simulink model "controller"  (R2020a)
settings: Solver=FixedStepDiscrete  StartTime=0.0  StopTime=10.0  FixedStep=0.01  MaxStep=0.01  RelTol=1e-3
undefined symbols (not defined in the file): DiscIntNeverNeededParam
libraries: dspfdesign x2, powerlib_meascontrol x2, simulink x2, dspswit3 x1, dspsigattribs x1
Description:
  | Ventilator Controller
settings Model: Creator=upattacini  LastModifiedBy=upattacini
settings SolverCC: MaxConsecutiveMinStep=10
settings DataIOCC: SaveOutput=off  SignalLogging=off  DSMLogging=off  SaveTime=off  ReturnWorkspaceOutputs=off
settings OptimizationCC: DefaultUnderspecifiedDataType=single  StrengthReduction=on  ZeroExternalMemoryAtStartup=off  ZeroInternalMemoryAtStartup=off  OptimizeBlockOrder=speed  OptimizationPriority=Speed  OptimizationCustomize=off  MultiThreadedLoops=on  EfficientTunableParamExpr=on
settings DebuggingCC: ParameterTunabilityLossMsg=error
settings SFSimCC: MATLABDynamicMemAlloc=off
settings RTWCC: SystemTargetFile=ert.tlc  GenCodeOnly=on  PackageGeneratedCodeAndArtifacts=on  PackageName=controller  TemplateMakefile=ert_default_tmf  TargetLang=C++
settings CodeAppCC: ForceParamTrailComments=on  IgnoreCustomStorageClasses=off  OperatorAnnotations=on  SimulinkDataObjDesc=on  SFDataObjDesc=on  InsertBlockDesc=on
settings ERTTargetCC: TargetLangStandard=C++03 (ISO)  GenerateSampleERTMain=on  MultiInstanceERTCode=on  CodeInterfacePackaging=C++ class  RootIOFormat=Structure reference  ERTCustomFileTemplate=example_file_process.tlc

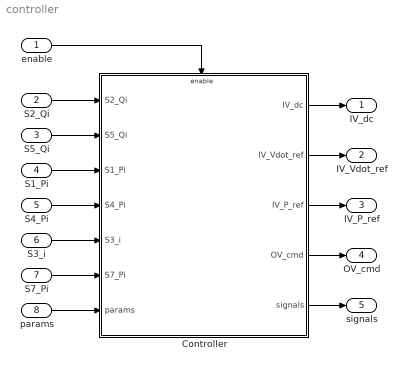
== system controller ==
  enable : Inport  OutDataTypeStr=boolean
  S2_Qi : Inport  Port=2  OutDataTypeStr=single
  S5_Qi : Inport  Port=3  OutDataTypeStr=single
  S1_Pi : Inport  Port=4  OutDataTypeStr=single
  S4_Pi : Inport  Port=5  OutDataTypeStr=single
  S3_i : Inport  Port=6  OutDataTypeStr=single  PortDimensions=2
  S7_Pi : Inport  Port=7  OutDataTypeStr=single
  params : Inport  Port=8  OutDataTypeStr=single  PortDimensions=3
  Controller : Subsystem  Tag=PublishSubsystem  mask(Controller){control_mode=PRESSURE, tidal_volume=0.65, PIP=35, PIP_step_perc=75, PIP_rise_perc=70, PEEP=5, respiratory_rate=10, IE_ratio=1/2, VC_P=0.2, VC_I=10, PC_FFW=30, PC_P=1, PC_I=40, HSC_cutoff=25, enable_trigger=off, trigger_inhibition_time=0.5, trigger_cutoff=2.5, trigger_filtder_tau=0.1, trigger_hyst_up=-5, trigger_hyst_down=-10}
      mask prompts: control_mode "Control Mode"; tidal_volume "Tidal Volume (L)"; PIP "PIP (cmH2O)"; PIP_step_perc "PIP Step Percentage (%)"; PIP_rise_perc "PIP Rising Percentage (%)"; PEEP "PEEP (cmH2O)"; respiratory_rate "Respiratory Rate (breaths/min)"; IE_ratio "Inspiration to Expiration Ratio"; VC_P "Proportional (%FS/SLPM)"; VC_I "Integral (%FS/(SLPM*s))"; PC_FFW "Feed-Forward (%FS)"; PC_P "Proportional (%FS/cmH2O)"; PC_I "Integral (%FS/(cmH2O*s))"; HSC_cutoff "HSC Cutoff Frequency (Hz)"; enable_trigger "Enable Triggering"; trigger_inhibition_time "Inhibition Time (s)"; trigger_cutoff "S3 Cutoff Frequency (Hz)"; trigger_filtder_tau "Derivative Filter Time Constant (s)"; trigger_hyst_up "Hysteresis Threshold Up (cmH2O/s)"; trigger_hyst_down "Hysteresis Threshold Down (cmH2O/s)"
      mask help: The controller generates the input signals that controls the inspiratory flow and expiratory valve.
      mask init:
      | Ts = eval(get_param(gcs, 'FixedStep'));
      | 
      | VC_mode = control_mode == 2;
      | PC_mode = control_mode == 3;
      | 
      | PC_IST = (IE_ratio/(IE_ratio+1) * (60 / respiratory_rate)) * (PIP_rise_perc/100) / 1.5;
      | a = -150.7658/(PC_IST*PC_IST*PC_IST);
      | b = -84.98128/(PC_IST*PC_IST);
      | c = -15.96696/PC_IST;
      | 
      | m = 4.0*c*Ts;
      | n = 2.0*b*Ts*Ts;
      | p = a*Ts*Ts*Ts;
      | 
      | PC_IST_num = [p, 3*p, 3*p, p];
      | PC_IST_den = [m+n+p-8, -m+n+3*p+24, -m-n+3*p-24, m-n+p+8];
      | PC_IST_x0_Gain = (PC_IST_den(2) - PC_IST_num(1)) / ...
      |                  ( PC_IST_num(2)*sum(PC_IST_den(2:end)) + ...
      |                  PC_IST_den(2)*sum(PC_IST_num(2:end)) );
      mask TypeOptions control_mode: OFF | VOLUME | PRESSURE
      mask Callback control_mode:
      | numparams = Simulink.Mask.get(gcb).numParameters;
      | enable = cell(1, numparams);
      | enable(:) = {'on'};
      | 
      | control_mode = get_param(gcb, 'control_mode');
      | if strcmpi(control_mode, 'VOLUME')
      |     enable(3:5) = {'off'};
      |     enable(11:13) = {'off'};
      | elseif strcmpi(control_mode, 'PRESSURE')
      |     enable{2} = 'off';
      |     enable(9:10) = {'off'};
      | else
      |     enable(2:end-6) = {'off'};
      |     enable(end-4:end) = {'off'};
      | end
      | set_param(gcb, 'MaskEnables', enable);
      mask DialogControl Container2 Prompt: Medical Parameters
      mask DialogControl Container3 Prompt: Controller Parameters
      mask DialogControl Container4 Prompt: Volume Control
      mask DialogControl Container5 Prompt: Pressure Control
      mask DialogControl Container6 Prompt: Filtering
      mask DialogControl Container7 Prompt: Assisted Ventilation
  IV_dc : Outport
  IV_Vdot_ref : Outport  Port=2
  IV_P_ref : Outport  Port=3
  OV_cmd : Outport  Port=4
  signals : Outport  Port=5
  wires:
  S2_Qi/1 -> Controller/1(S2_Qi)
  Controller/1(IV_dc) -> IV_dc/1
  Controller/2(IV_Vdot_ref) -> IV_Vdot_ref/1
  Controller/4(OV_cmd) -> OV_cmd/1
  S1_Pi/1 -> Controller/3(S1_Pi)
  Controller/3(IV_P_ref) -> IV_P_ref/1
  Controller/5(signals) -> signals/1
  enable/1 -> Controller/Enable
  S5_Qi/1 -> Controller/2(S5_Qi)
  S4_Pi/1 -> Controller/4(S4_Pi)
  params/1 -> Controller/7(params)
  S3_i/1 -> Controller/5(S3_i)
  S7_Pi/1 -> Controller/6(S7_Pi)

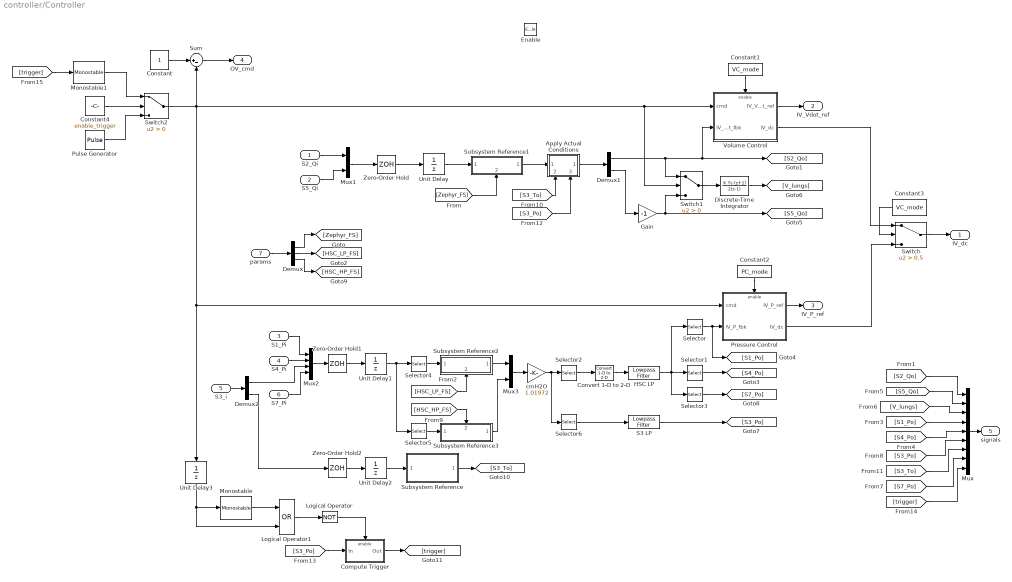
== system controller/Controller ==
  S2_Qi : Inport
  S5_Qi : Inport  Port=2
  S1_Pi : Inport  Port=3
  S4_Pi : Inport  Port=4
  S3_i : Inport  Port=5
  S7_Pi : Inport  Port=6
  params : Inport  Port=7
  Enable : EnablePort  StatesWhenEnabling=reset
  Apply Actual Conditions : Subsystem  ReferencedSubsystem=apply_actual_conditions
      settings: PortSchema="{\"entries\":[{\"content\":{\"sides\":[{\"content\":{\"connectorIds\":[\"In1\"]},\"type\":\"ConnectorPlacement.EquallySpacedRectSide\",\"uuid\":\"3b4e15f5-ec7a-455d-a112-e063b421ee9f\"},{\"content\":{\"connectorIds\":[\"Out1\"],\"side\":\"RIGHT\"},\"type\":\"ConnectorPlacement.EquallySpacedRectSide\",\"uuid\":\"595b3fd5-6603-4191-b183-4edf5336d9a2\"},{\"content\":{\"connectorIds\":[],\"side\":\"TOP\"},\"type\":\"ConnectorPlacement.EquallySpacedRectSide\",\"uuid\":\"7211f4ea-7225-4536-b1e6-5aea95971c19\"},{\"content\":{\"connectorIds\":[\"In2\",\"In3\"],\"side\":\"BOTTOM\"},\"type\":\"ConnectorPlacement.EquallySpacedRectSide\",\"uuid\":\"c060314b-2654-4a54-a68c-60767f6efbb5\"}]},\"type\":\"ConnectorPlacement.EquallySpacedConnector\",\"uuid\":\"0e2934c3-16fd-4aed-85e0-c12757e58969\"}],\"packageUris\":[\"http://schema.mathworks.com/mf0/Connector/19700101\"],\"version\":\"1.0\"}"
  Compute Trigger : Subsystem
  Constant : Constant  OutDataTypeStr=single
  Constant1 : Constant  Value=VC_mode
  Constant2 : Constant  Value=PC_mode
  Constant3 : Constant  Value=VC_mode
  Constant4 : Constant  Value=enable_trigger  OutDataTypeStr=boolean
  Convert 1-D to 2-D : dspsigattribs/Convert 1-D to 2-D  M=1  N=3  frameBasedOut=off
      settings: SourceProductBaseCode=DS
  Demux : Demux  Outputs=3
  Demux1 : Demux  Outputs=2
  Demux2 : Demux  Outputs=2
  Discrete-Time Integrator : DiscreteIntegrator  IntegratorMethod=Integration: Trapezoidal  gainval=1/60  SampleTime=-1  ICPrevOutput=DiscIntNeverNeededParam  ICPrevScaledInput=DiscIntNeverNeededParam
  Gain : Gain  Gain=-1
  HSC LP : dspfdesign/Lowpass Filter  FilterType=IIR  DesignForMinimumOrder=off  FilterOrder=3  PassbandFrequency=HSC_cutoff  StopbandFrequency=12e3  PassbandRipple=0.5  StopbandAttenuation=30  InheritSampleRate=on  SampleRate=44100  SimulateUsing=Code generation  roundingMode=Floor  coeffsDataTypeStr=fixdt(1,16)
  Logical Operator : Logic  Operator=NOT  AllPortsSameDT=off  OutDataTypeStr=boolean
  Logical Operator1 : Logic  Operator=OR  AllPortsSameDT=off  OutDataTypeStr=boolean
  Monostable : powerlib_meascontrol/Logic/Monostable  EdgeDetect=Falling  PulseDuration=trigger_inhibition_time  ic=0  Ts=Ts
      settings: SourceProductBaseCode=PS
  Monostable1 : powerlib_meascontrol/Logic/Monostable  EdgeDetect=Rising  PulseDuration=IE_ratio/(IE_ratio+1) * (60 / respiratory_rate)  ic=0  Ts=Ts
      settings: SourceProductBaseCode=PS
  Mux : Mux  Inputs=9
  Mux1 : Mux  Inputs=2
  Mux2 : Mux
  Mux3 : Mux  Inputs=2
  Pressure Control : Subsystem
  Pulse Generator : DiscretePulseGenerator  Period=floor((60 / respiratory_rate) / Ts)  PulseWidth=floor((IE_ratio/(IE_ratio+1) * (60 / respiratory_rate)) / Ts)  SampleTime=Ts
  S3 LP : dspfdesign/Lowpass Filter  FilterType=IIR  DesignForMinimumOrder=off  FilterOrder=3  PassbandFrequency=trigger_cutoff  StopbandFrequency=12e3  PassbandRipple=0.5  StopbandAttenuation=30  InheritSampleRate=on  SampleRate=44100  SimulateUsing=Code generation  roundingMode=Floor  coeffsDataTypeStr=fixdt(1,16)
  Selector : Selector  InputPortWidth=3  IndexOptions=Index vector (dialog)  Indices=1  OutputSizes=1
  Selector1 : Selector  InputPortWidth=3  IndexOptions=Index vector (dialog)  Indices=2  OutputSizes=1
  Selector2 : Selector  InputPortWidth=4  IndexOptions=Index vector (dialog)  Indices=[1 2 4]  OutputSizes=1
  Selector3 : Selector  InputPortWidth=3  IndexOptions=Index vector (dialog)  Indices=3  OutputSizes=1
  Selector4 : Selector  InputPortWidth=4  IndexOptions=Index vector (dialog)  Indices=[1 2 3]  OutputSizes=1
  Selector5 : Selector  InputPortWidth=4  IndexOptions=Index vector (dialog)  Indices=4  OutputSizes=1
  Selector6 : Selector  InputPortWidth=4  IndexOptions=Index vector (dialog)  Indices=3  OutputSizes=1
  Subsystem Reference : Subsystem  ReferencedSubsystem=T_decoder
  Subsystem Reference1 : Subsystem  ReferencedSubsystem=HSC_decoder
      settings: PortSchema="{\"entries\":[{\"content\":{\"sides\":[{\"content\":{\"connectorIds\":[\"In1\"]},\"type\":\"ConnectorPlacement.EquallySpacedRectSide\",\"uuid\":\"71a4e4f9-9ef6-4add-947e-0b57a706a0fc\"},{\"content\":{\"connectorIds\":[\"Out1\"],\"side\":\"RIGHT\"},\"type\":\"ConnectorPlacement.EquallySpacedRectSide\",\"uuid\":\"d997839f-7697-403c-ab31-97bb95e5d26f\"},{\"content\":{\"connectorIds\":[],\"side\":\"TOP\"},\"type\":\"ConnectorPlacement.EquallySpacedRectSide\",\"uuid\":\"6a2eaf4c-1277-4d90-b513-5efc8abce9b0\"},{\"content\":{\"connectorIds\":[\"In2\"],\"side\":\"BOTTOM\"},\"type\":\"ConnectorPlacement.EquallySpacedRectSide\",\"uuid\":\"a341bd79-bd1c-4a8b-9abf-5623b4073918\"}]},\"type\":\"ConnectorPlacement.EquallySpacedConnector\",\"uuid\":\"c1361fad-ebea-4dab-bf9b-dc7c859591e9\"}],\"packageUris\":[\"http://schema.mathworks.com/mf0/Connector/19700101\"],\"version\":\"1.0\"}"
  Subsystem Reference2 : Subsystem  ReferencedSubsystem=HSC_decoder
      settings: PortSchema="{\"entries\":[{\"content\":{\"sides\":[{\"content\":{\"connectorIds\":[\"In1\"]},\"type\":\"ConnectorPlacement.EquallySpacedRectSide\",\"uuid\":\"71a4e4f9-9ef6-4add-947e-0b57a706a0fc\"},{\"content\":{\"connectorIds\":[\"Out1\"],\"side\":\"RIGHT\"},\"type\":\"ConnectorPlacement.EquallySpacedRectSide\",\"uuid\":\"d997839f-7697-403c-ab31-97bb95e5d26f\"},{\"content\":{\"connectorIds\":[],\"side\":\"TOP\"},\"type\":\"ConnectorPlacement.EquallySpacedRectSide\",\"uuid\":\"6a2eaf4c-1277-4d90-b513-5efc8abce9b0\"},{\"content\":{\"connectorIds\":[\"In2\"],\"side\":\"BOTTOM\"},\"type\":\"ConnectorPlacement.EquallySpacedRectSide\",\"uuid\":\"a341bd79-bd1c-4a8b-9abf-5623b4073918\"}]},\"type\":\"ConnectorPlacement.EquallySpacedConnector\",\"uuid\":\"c1361fad-ebea-4dab-bf9b-dc7c859591e9\"}],\"packageUris\":[\"http://schema.mathworks.com/mf0/Connector/19700101\"],\"version\":\"1.0\"}"
  Subsystem Reference3 : Subsystem  ReferencedSubsystem=HSC_decoder
      settings: PortSchema="{\"entries\":[{\"content\":{\"sides\":[{\"content\":{\"connectorIds\":[\"In1\"]},\"type\":\"ConnectorPlacement.EquallySpacedRectSide\",\"uuid\":\"71a4e4f9-9ef6-4add-947e-0b57a706a0fc\"},{\"content\":{\"connectorIds\":[\"Out1\"],\"side\":\"RIGHT\"},\"type\":\"ConnectorPlacement.EquallySpacedRectSide\",\"uuid\":\"d997839f-7697-403c-ab31-97bb95e5d26f\"},{\"content\":{\"connectorIds\":[\"In2\"],\"side\":\"TOP\"},\"type\":\"ConnectorPlacement.EquallySpacedRectSide\",\"uuid\":\"6a2eaf4c-1277-4d90-b513-5efc8abce9b0\"},{\"content\":{\"connectorIds\":[],\"side\":\"BOTTOM\"},\"type\":\"ConnectorPlacement.EquallySpacedRectSide\",\"uuid\":\"a341bd79-bd1c-4a8b-9abf-5623b4073918\"}]},\"type\":\"ConnectorPlacement.EquallySpacedConnector\",\"uuid\":\"c1361fad-ebea-4dab-bf9b-dc7c859591e9\"}],\"packageUris\":[\"http://schema.mathworks.com/mf0/Connector/19700101\"],\"version\":\"1.0\"}"
  Sum : Sum  Inputs=|+-
  Switch : Switch  Criteria=u2 > Threshold  Threshold=0.5
  Switch1 : Switch  Criteria=u2 > Threshold
  Switch2 : Switch  Criteria=u2 > Threshold  OutDataTypeStr=single
  Unit Delay : UnitDelay  SampleTime=-1  HasFrameUpgradeWarning=on
  Unit Delay1 : UnitDelay  InitialCondition=0.1 * 16384  SampleTime=-1  HasFrameUpgradeWarning=on
  Unit Delay2 : UnitDelay  SampleTime=-1  HasFrameUpgradeWarning=on
  Unit Delay3 : UnitDelay  SampleTime=-1  HasFrameUpgradeWarning=on
  Volume Control : Subsystem
  Zero-Order Hold : ZeroOrderHold  SampleTime=Ts
  Zero-Order Hold1 : ZeroOrderHold  SampleTime=Ts
  Zero-Order Hold2 : ZeroOrderHold  SampleTime=Ts
  cmH2O : Gain  Gain=1.01972
  IV_dc : Outport  OutputWhenDisabled=reset  InitialOutput=0
  IV_Vdot_ref : Outport  Port=2  OutputWhenDisabled=reset  InitialOutput=0
  IV_P_ref : Outport  Port=3  OutputWhenDisabled=reset  InitialOutput=0
  OV_cmd : Outport  Port=4  OutputWhenDisabled=reset  InitialOutput=0
  signals : Outport  Port=5  OutputWhenDisabled=reset  InitialOutput=0
  wires:
  Constant/1 -> Sum/1
  Sum/1 -> OV_cmd/1
  Volume Control/1(IV_Vdot_ref) -> IV_Vdot_ref/1
  Constant1/1 -> Volume Control/Enable
  Constant2/1 -> Pressure Control/Enable
  Switch/1 -> IV_dc/1
  Volume Control/2(IV_dc) -> Switch/1
  Pressure Control/2(IV_dc) -> Switch/3
  Constant3/1 -> Switch/2
  Pressure Control/1(IV_P_ref) -> IV_P_ref/1
  params/1 -> Demux/1
  Demux/1 -> [Zephyr_FS]
  [Zephyr_FS] -> Subsystem Reference1/2
  [S2_Qo] -> Mux/1
  Mux/1 -> signals/1
  Zero-Order Hold/1 -> Unit Delay/1
  Zero-Order Hold1/1 -> Unit Delay1/1
  Unit Delay1/1 -> Selector5/1, Selector4/1
  Demux/2 -> [HSC_LP_FS]
  [HSC_LP_FS] -> Subsystem Reference2/2
  [S5_Qo] -> Mux/2
  Gain/1 -> Switch1/3, [S5_Qo]
  [S1_Po] -> Mux/4
  [S4_Po] -> Mux/5
  Discrete-Time Integrator/1 -> [V_lungs]
  [V_lungs] -> Mux/3
  [S3_Po] -> Mux/6
  S2_Qi/1 -> Mux1/1
  S5_Qi/1 -> Mux1/2
  Mux1/1 -> Zero-Order Hold/1
  S4_Pi/1 -> Mux2/2
  Mux2/1 -> Zero-Order Hold1/1
  Convert 1-D to 2-D/1 -> HSC LP/1
  Selector/1 -> [S1_Po], Pressure Control/2(IV_P_fbk)
  HSC LP/1 -> Selector3/1, Selector1/1, Selector/1
  Selector1/1 -> [S4_Po]
  S7_Pi/1 -> Mux2/4
  Selector3/1 -> [S7_Po]
  Demux/3 -> [HSC_HP_FS]
  Selector4/1 -> Subsystem Reference2/1
  Selector5/1 -> Subsystem Reference3/1
  [HSC_HP_FS] -> Subsystem Reference3/2
  Subsystem Reference2/1 -> Mux3/1
  Subsystem Reference3/1 -> Mux3/2
  Mux3/1 -> cmH2O/1
  S1_Pi/1 -> Mux2/1
  Demux2/1 -> Mux2/3
  [S7_Po] -> Mux/8
  Demux2/2 -> Zero-Order Hold2/1
  S3_i/1 -> Demux2/1
  Demux1/1 -> Switch1/1, Volume Control/2(IV_Vdot_fbk), [S2_Qo]
  Demux1/2 -> Gain/1
  Unit Delay2/1 -> Subsystem Reference/1
  [S3_To] -> Mux/7
  Zero-Order Hold2/1 -> Unit Delay2/1
  Subsystem Reference/1 -> [S3_To]
  [S3_To] -> Apply Actual Conditions/2
  Unit Delay/1 -> Subsystem Reference1/1
  Subsystem Reference1/1 -> Apply Actual Conditions/1
  Apply Actual Conditions/1 -> Demux1/1
  Switch1/1 -> Discrete-Time Integrator/1
  [trigger] -> Mux/9
  Compute Trigger/1(Out) -> [trigger]
  Monostable/1 -> Logical Operator1/1
  Logical Operator1/1 -> Logical Operator/1
  Constant4/1 -> Switch2/2
  Pulse Generator/1 -> Switch2/3
  Logical Operator/1 -> Compute Trigger/Enable
  Unit Delay3/1 -> Logical Operator1/2, Monostable/1
  Monostable1/1 -> Switch2/1
  Switch2/1 -> Switch1/2, Volume Control/1(cmd), Pressure Control/1(cmd), Unit Delay3/1, Sum/2
  [trigger] -> Monostable1/1
  cmH2O/1 -> Selector6/1, Selector2/1
  [S3_Po] -> Apply Actual Conditions/3
  [S3_Po] -> Compute Trigger/1(In)
  Selector2/1 -> Convert 1-D to 2-D/1
  Selector6/1 -> S3 LP/1
  S3 LP/1 -> [S3_Po]

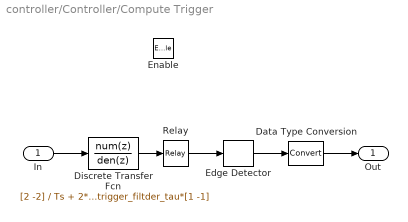
== system controller/Controller/Compute Trigger ==
  In : Inport
  Enable : EnablePort  StatesWhenEnabling=reset
  Data Type Conversion : DataTypeConversion
  Discrete Transfer Fcn : DiscreteTransferFcn  Numerator=[2 -2]  Denominator=Ts + 2*trigger_filtder_tau*[1 -1]
  Edge Detector : dspswit3/Edge Detector  InputProcessing=Columns as channels (frame based)
      settings: SourceProductBaseCode=DS
  Relay : Relay  OnSwitchValue=trigger_hyst_up  OffSwitchValue=trigger_hyst_down  OnOutputValue=0  OffOutputValue=1  OutDataTypeStr=Inherit: Inherit via back propagation
  Out : Outport  OutputWhenDisabled=reset  InitialOutput=0
  wires:
  Relay/1 -> Edge Detector/1
  Edge Detector/1 -> Data Type Conversion/1
  Data Type Conversion/1 -> Out/1
  Discrete Transfer Fcn/1 -> Relay/1
  In/1 -> Discrete Transfer Fcn/1

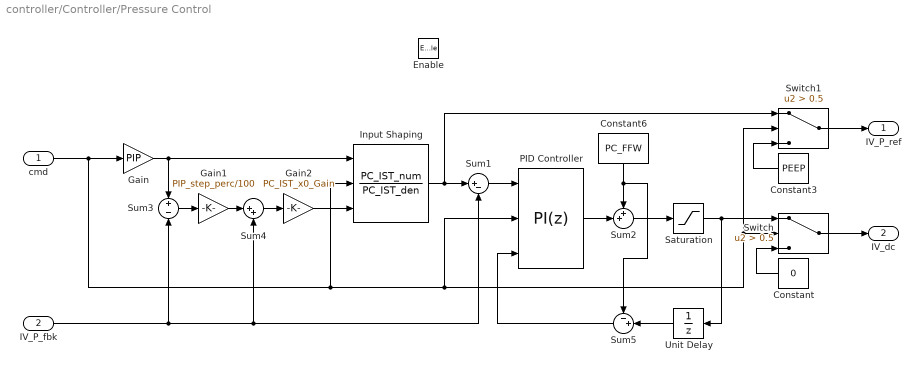
== system controller/Controller/Pressure Control ==
  cmd : Inport
  IV_P_fbk : Inport  Port=2
  Enable : EnablePort  StatesWhenEnabling=reset
  Constant : Constant  Value=0  OutDataTypeStr=single
  Constant3 : Constant  Value=PEEP  OutDataTypeStr=single
  Constant6 : Constant  Value=PC_FFW  OutDataTypeStr=single
  Gain : Gain  Gain=PIP
  Gain1 : Gain  Gain=PIP_step_perc/100
  Gain2 : Gain  Gain=PC_IST_x0_Gain
  Input Shaping : DiscreteFilter  Numerator=PC_IST_num  Denominator=PC_IST_den  InitialStatesSource=Input port  ExternalReset=Rising
      settings: InputPortMap=u0,r7,p5
  PID Controller : simulink/Continuous/PID Controller  Controller=PI  Form=Parallel  TimeDomain=Discrete-time  UseExternalTs=off  SampleTime=-1  IntegratorMethod=Trapezoidal  FilterMethod=Trapezoidal  ControllerParametersSource=internal  P=PC_P  I=PC_I  D=1  UseFilter=on  N=100  TunerSelectOption=Transfer Function Based (PID Tuner App)  InitialConditionSource=internal  InitialConditionForIntegrator=0  InitialConditionForFilter=0  DifferentiatorICPrevScaledInput=0  ExternalReset=rising  TrackingMode=on  Kt=1  LimitOutput=off  UpperSaturationLimit=100  LowerSaturationLimit=0  LinearizeAsGain=on  AntiWindupMode=clamping  Kb=1  POutMin=[]  POutMax=[]  IOutMin=[]  IOutMax=[]  DOutMin=[]  DOutMax=[]  NOutMin=[]  NOutMax=[]  SumOutMin=[]  SumOutMax=[]  SaturationOutMin=[]  SaturationOutMax=[]  PParamMin=[]  PParamMax=[]  IParamMin=[]  IParamMax=[]  DParamMin=[]  DParamMax=[]  NParamMin=[]  NParamMax=[]  KbParamMin=[]  KbParamMax=[]  KtParamMin=[]  KtParamMax=[]  KbOutMin=[]  KbOutMax=[]  KtOutMin=[]  KtOutMax=[]  IntegratorOutMin=[]  IntegratorOutMax=[]  FilterOutMin=[]  FilterOutMax=[]  SumI1OutMin=[]  SumI1OutMax=[]  SumI2OutMin=[]  SumI2OutMax=[]  SumI3OutMin=[]  SumI3OutMax=[]  SumI4OutMin=[]  SumI4OutMax=[]  SumDOutMin=[]  SumDOutMax=[]  DifferentiatorOutMin=[]  DifferentiatorOutMax=[]  FilterDiffOutCoefMin=[]  FilterDiffOutCoefMax=[]  ReciprocalOutMin=[]  ReciprocalOutMax=[]  SumDenOutMin=[]  SumDenOutMax=[]  SumNumOutMin=[]  SumNumOutMax=[]  DivideOutMin=[]  DivideOutMax=[]  UdiffTsProdOutMin=[]  UdiffTsProdOutMax=[]  NTsProdOutMin=[]  NTsProdOutMax=[]  UintegralTsProdOutMin=[]  UintegralTsProdOutMax=[]  UngainTsProdOutMin=[]  UngainTsProdOutMax=[]  IntegratorContinuousStateAttributes=''  IntegratorStateMustResolveToSignalObject=off  IntegratorRTWStateStorageClass=Auto  FilterContinuousStateAttributes=''  FilterStateMustResolveToSignalObject=off  FilterRTWStateStorageClass=Auto  ParallelPVariant=InternalParameters  IdealPVariant=Disabled  IVariant=InternalParameters  DVariant=Disabled  IntegratorVariant=Discrete  SatVariant=Disabled  AWVariant=Passthrough  PCopyVariant=Disabled  TRVariant=Enabled  FdbkBlocksVariant=Feedback  IdealPFdbkVariant=Passthrough  SatFdbkVariant=Passthrough  DerivativeFilterVariant=Disabled  NVariant=Disabled  NCopyVariant=Disabled_SignalSpec  FilterICVariant=Disabled  IntegratorICVariant=InternalICs  ExternalResetVariant=ExternalReset  TRSumVariant=TrackingMode  SumFdbkVariant=Enabled  SumVariant=Sum_PI  TsampFilterVariant=InternalTs  TsampNgainVariant=Passthrough  TsampIntegralVariant=Passthrough
  Saturation : Saturate  UpperLimit=100  LowerLimit=0
  Sum1 : Sum  Inputs=|+-
  Sum2 : Sum  Inputs=++|
  Sum3 : Sum  Inputs=+-
  Sum4 : Sum  Inputs=|++
  Sum5 : Sum  Inputs=-+|
  Switch : Switch  Criteria=u2 > Threshold  Threshold=0.5
  Switch1 : Switch  Criteria=u2 > Threshold  Threshold=0.5
  Unit Delay : UnitDelay  SampleTime=-1  HasFrameUpgradeWarning=on
  IV_P_ref : Outport  OutputWhenDisabled=reset  InitialOutput=0
  IV_dc : Outport  Port=2  OutputWhenDisabled=reset  InitialOutput=0
  wires:
  Sum1/1 -> PID Controller/1
  Saturation/1 -> Switch/1, Unit Delay/1
  Switch/1 -> IV_dc/1
  Constant/1 -> Switch/3
  Switch1/1 -> IV_P_ref/1
  Gain/1 -> Input Shaping/1, Sum3/1
  Constant3/1 -> Switch1/3
  IV_P_fbk/1 -> Sum3/2, Sum4/2, Sum1/2
  PID Controller/1 -> Sum2/2
  Sum2/1 -> Saturation/1
  cmd/1 -> Input Shaping/2, PID Controller/2, Switch1/2, Switch/2, Gain/1
  Input Shaping/1 -> Switch1/1, Sum1/1
  Constant6/1 -> Sum5/1, Sum2/1
  Sum3/1 -> Gain1/1
  Gain2/1 -> Input Shaping/3
  Gain1/1 -> Sum4/1
  Sum4/1 -> Gain2/1
  Sum5/1 -> PID Controller/3
  Unit Delay/1 -> Sum5/2

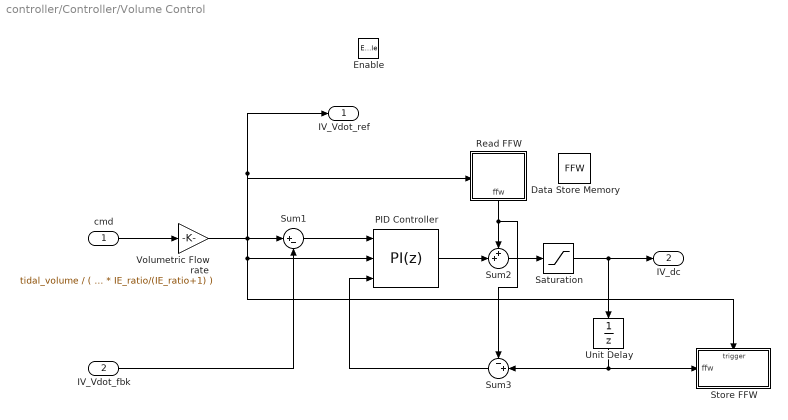
== system controller/Controller/Volume Control ==
  cmd : Inport
  IV_Vdot_fbk : Inport  Port=2
  Enable : EnablePort  StatesWhenEnabling=reset
  Data Store Memory : DataStoreMemory  DataStoreName=FFW  ReadBeforeWriteMsg=warning  WriteAfterWriteMsg=warning  WriteAfterReadMsg=warning  ShowAdditionalParam=off  OutMin=0  OutMax=100
  PID Controller : simulink/Continuous/PID Controller  Controller=PI  Form=Parallel  TimeDomain=Discrete-time  UseExternalTs=off  SampleTime=-1  IntegratorMethod=Trapezoidal  FilterMethod=Forward Euler  ControllerParametersSource=internal  P=VC_P  I=VC_I  D=1  UseFilter=on  N=100  TunerSelectOption=Transfer Function Based (PID Tuner App)  InitialConditionSource=internal  InitialConditionForIntegrator=0  InitialConditionForFilter=0  DifferentiatorICPrevScaledInput=0  ExternalReset=falling  TrackingMode=on  Kt=1  LimitOutput=off  UpperSaturationLimit=100  LowerSaturationLimit=0  LinearizeAsGain=on  AntiWindupMode=clamping  Kb=1  POutMin=[]  POutMax=[]  IOutMin=[]  IOutMax=[]  DOutMin=[]  DOutMax=[]  NOutMin=[]  NOutMax=[]  SumOutMin=[]  SumOutMax=[]  SaturationOutMin=[]  SaturationOutMax=[]  PParamMin=[]  PParamMax=[]  IParamMin=[]  IParamMax=[]  DParamMin=[]  DParamMax=[]  NParamMin=[]  NParamMax=[]  KbParamMin=[]  KbParamMax=[]  KtParamMin=[]  KtParamMax=[]  KbOutMin=[]  KbOutMax=[]  KtOutMin=[]  KtOutMax=[]  IntegratorOutMin=[]  IntegratorOutMax=[]  FilterOutMin=[]  FilterOutMax=[]  SumI1OutMin=[]  SumI1OutMax=[]  SumI2OutMin=[]  SumI2OutMax=[]  SumI3OutMin=[]  SumI3OutMax=[]  SumI4OutMin=[]  SumI4OutMax=[]  SumDOutMin=[]  SumDOutMax=[]  DifferentiatorOutMin=[]  DifferentiatorOutMax=[]  FilterDiffOutCoefMin=[]  FilterDiffOutCoefMax=[]  ReciprocalOutMin=[]  ReciprocalOutMax=[]  SumDenOutMin=[]  SumDenOutMax=[]  SumNumOutMin=[]  SumNumOutMax=[]  DivideOutMin=[]  DivideOutMax=[]  UdiffTsProdOutMin=[]  UdiffTsProdOutMax=[]  NTsProdOutMin=[]  NTsProdOutMax=[]  UintegralTsProdOutMin=[]  UintegralTsProdOutMax=[]  UngainTsProdOutMin=[]  UngainTsProdOutMax=[]  IntegratorContinuousStateAttributes=''  IntegratorStateMustResolveToSignalObject=off  IntegratorRTWStateStorageClass=Auto  FilterContinuousStateAttributes=''  FilterStateMustResolveToSignalObject=off  FilterRTWStateStorageClass=Auto  ParallelPVariant=InternalParameters  IdealPVariant=Disabled  IVariant=InternalParameters  DVariant=Disabled  IntegratorVariant=Discrete  SatVariant=Disabled  AWVariant=Passthrough  PCopyVariant=Disabled  TRVariant=Enabled  FdbkBlocksVariant=Feedback  IdealPFdbkVariant=Passthrough  SatFdbkVariant=Passthrough  DerivativeFilterVariant=Disabled  NVariant=Disabled  NCopyVariant=Disabled_SignalSpec  FilterICVariant=Disabled  IntegratorICVariant=InternalICs  ExternalResetVariant=ExternalReset  TRSumVariant=TrackingMode  SumFdbkVariant=Enabled  SumVariant=Sum_PI  TsampFilterVariant=InternalTs  TsampNgainVariant=Passthrough  TsampIntegralVariant=Passthrough
  Read FFW : Subsystem  TreatAsAtomicUnit=on
  Saturation : Saturate  UpperLimit=100  LowerLimit=0
  Store FFW : Subsystem  TreatAsAtomicUnit=on
  Sum1 : Sum  Inputs=|+-
  Sum2 : Sum  Inputs=++|
  Sum3 : Sum  Inputs=-+|
  Unit Delay : UnitDelay  SampleTime=-1  HasFrameUpgradeWarning=on
  Volumetric Flow rate : Gain  Gain=tidal_volume / ( (1/respiratory_rate) * IE_ratio/(IE_ratio+1) )
  IV_Vdot_ref : Outport  OutputWhenDisabled=reset  InitialOutput=0
  IV_dc : Outport  Port=2  OutputWhenDisabled=reset  InitialOutput=0
  wires:
  Read FFW/1(ffw) -> Sum3/1, Sum2/1
  Volumetric Flow rate/1 -> PID Controller/2, Store FFW/Trigger, Sum1/1, IV_Vdot_ref/1, Read FFW/Enable
  cmd/1 -> Volumetric Flow rate/1
  Sum2/1 -> Saturation/1
  Sum1/1 -> PID Controller/1
  PID Controller/1 -> Sum2/2
  Saturation/1 -> IV_dc/1, Unit Delay/1
  IV_Vdot_fbk/1 -> Sum1/2
  Sum3/1 -> PID Controller/3
  Unit Delay/1 -> Store FFW/1(ffw), Sum3/2

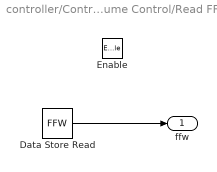
== system controller/Controller/Volume Control/Read FFW ==
  Enable : EnablePort
  Data Store Read : DataStoreRead  DataStoreName=FFW
  ffw : Outport  OutputWhenDisabled=reset  InitialOutput=0
  wires:
  Data Store Read/1 -> ffw/1

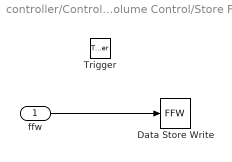
== system controller/Controller/Volume Control/Store FFW ==
  ffw : Inport
  Trigger : TriggerPort  TriggerType=falling  VariantControl=Variant  PortDimensions=1
  Data Store Write : DataStoreWrite  DataStoreName=FFW
  wires:
  ffw/1 -> Data Store Write/1
